simulink model "Week1_9"  (R2020b)
settings: Solver=VariableStepAuto  StartTime=0.0  StopTime=10.0  RelTol=1e-3
model workspace (MAT data in the model file):
  J = 0.01
  K = 0.01
  L = 0.5
  R = 1
  b = 0.1
settings Model: Creator=user  LastModifiedBy=user

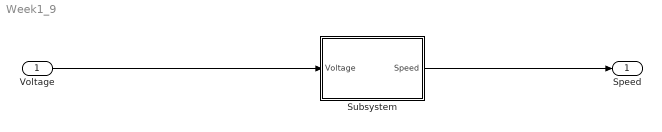
== system Week1_9 ==
  Voltage : Inport
  Subsystem : Subsystem
  Speed : Outport
  wires:
  Voltage/1 -> Subsystem/1(Voltage)
  Subsystem/1(Speed) -> Speed/1

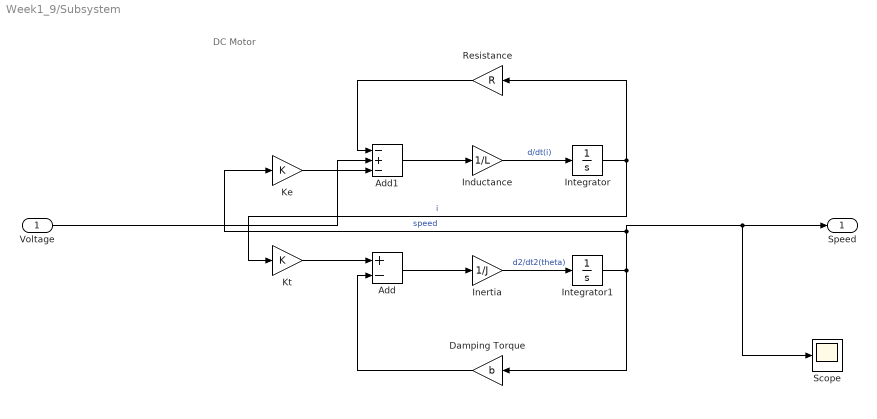
== system Week1_9/Subsystem ==
  note: DC Motor
  Voltage : Inport
  Add : Sum  Inputs=+-
  Add1 : Sum  Inputs=-+-
  Damping Torque : Gain  Gain=b
  Inductance : Gain  Gain=1/L
  Inertia : Gain  Gain=1/J
  Integrator : Integrator
  Integrator1 : Integrator
  Ke : Gain  Gain=K
  Kt : Gain  Gain=K
  Resistance : Gain  Gain=R
  Scope : Scope
  Speed : Outport
  wires:
  Add1/1 -> Inductance/1
  Ke/1 -> Add1/3
  Integrator/1 -> Kt/1, Resistance/1  "i"
  Integrator1/1 -> Speed/1, Scope/1, Ke/1, Damping Torque/1  "speed"
  Inertia/1 -> Integrator1/1  "d2/dt2(theta)"
  Damping Torque/1 -> Add/2
  Kt/1 -> Add/1
  Add/1 -> Inertia/1
  Resistance/1 -> Add1/1
  Voltage/1 -> Add1/2
  Inductance/1 -> Integrator/1  "d/dt(i)"
